simulink model "SimpleTC_SoftwareArch_SoftwareSystem_mapping"  (R2016a)
settings: Solver=FixedStepAuto  StartTime=0.0  StopTime=10.0  RelTol=1e-3
model workspace: external: MAT-File SimpleTC_SoftwareArch_SoftwareSystem_mapping.mat (data not in the file)
libraries: libTLAsserts x6, libAsserts x4
settings Model: Creator=Josef  LastModifiedBy=Josef
settings GRTTargetCC: GeneratePreprocessorConditionals=Use local settings

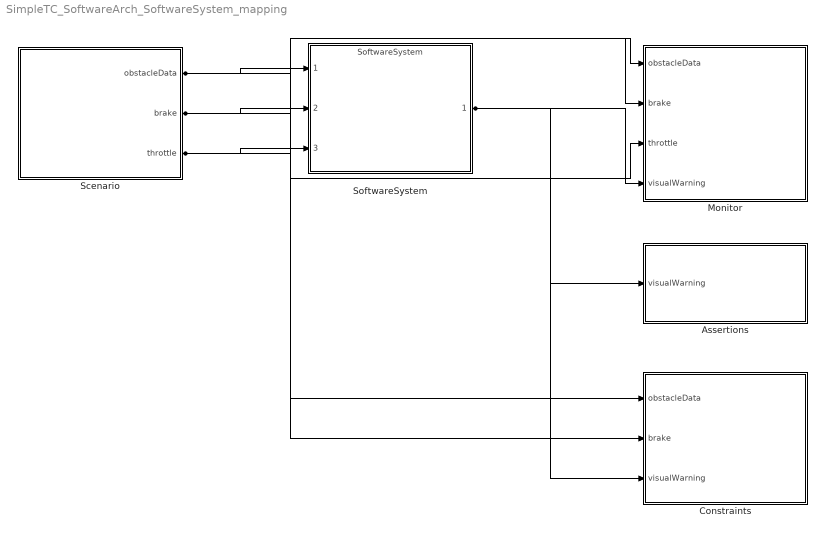
== system SimpleTC_SoftwareArch_SoftwareSystem_mapping ==
  Assertions : Subsystem
  Constraints : Subsystem
  Monitor : Subsystem
  Scenario : Subsystem
  SoftwareSystem : ModelReference  ModelNameDialog=SoftwareSystem  SimulationMode=Normal  ModelReferenceVersion=1.9
  wires:
  Scenario/2(brake) -> SoftwareSystem/2, Monitor/2(brake), Constraints/2(brake)
  Scenario/3(throttle) -> SoftwareSystem/3, Monitor/3(throttle)
  Scenario/1(obstacleData) -> SoftwareSystem/1, Monitor/1(obstacleData), Constraints/1(obstacleData)
  SoftwareSystem/1 -> Monitor/4(visualWarning), Assertions/1(visualWarning), Constraints/3(visualWarning)

== system SimpleTC_SoftwareArch_SoftwareSystem_mapping/Assertions ==
  visualWarning : Inport
  assert_1 : Subsystem
  simout_1 : ToFile  Filename=assert_1.mat  MatrixName=assert_1  SaveFormat=Timeseries
  wires:
  visualWarning/1 -> assert_1/1(visualWarning)
  assert_1/1(assert_1_FAILED) -> simout_1/1

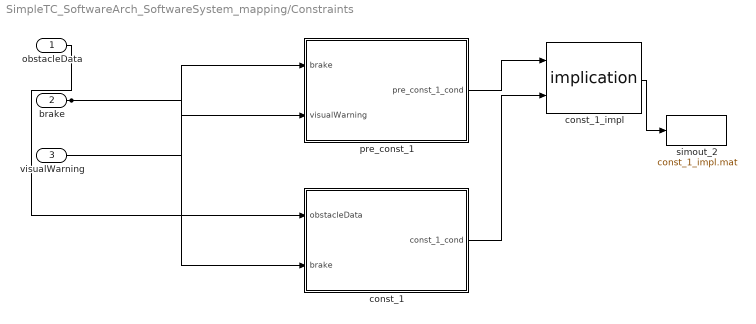
== system SimpleTC_SoftwareArch_SoftwareSystem_mapping/Constraints ==
  obstacleData : Inport
  brake : Inport  Port=2
  visualWarning : Inport  Port=3
  const_1 : Subsystem
  const_1_impl : libAsserts/implication
  pre_const_1 : Subsystem
  simout_2 : ToFile  Filename=const_1_impl.mat  MatrixName=const_1_impl  SaveFormat=Timeseries
  wires:
  brake/1 -> pre_const_1/1(brake), const_1/2(brake)
  visualWarning/1 -> pre_const_1/2(visualWarning)
  obstacleData/1 -> const_1/1(obstacleData)
  pre_const_1/1(pre_const_1_cond) -> const_1_impl/1
  const_1/1(const_1_cond) -> const_1_impl/2
  const_1_impl/1 -> simout_2/1

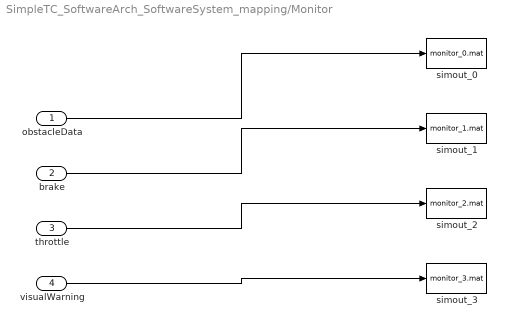
== system SimpleTC_SoftwareArch_SoftwareSystem_mapping/Monitor ==
  obstacleData : Inport
  brake : Inport  Port=2
  throttle : Inport  Port=3
  visualWarning : Inport  Port=4
  simout_0 : ToFile  Filename=monitor_0.mat  MatrixName=obstacleData  SaveFormat=Timeseries
  simout_1 : ToFile  Filename=monitor_1.mat  MatrixName=brake  SaveFormat=Timeseries
  simout_2 : ToFile  Filename=monitor_2.mat  MatrixName=throttle  SaveFormat=Timeseries
  simout_3 : ToFile  Filename=monitor_3.mat  MatrixName=visualWarning  SaveFormat=Timeseries
  wires:
  obstacleData/1 -> simout_0/1
  brake/1 -> simout_1/1
  throttle/1 -> simout_2/1
  visualWarning/1 -> simout_3/1

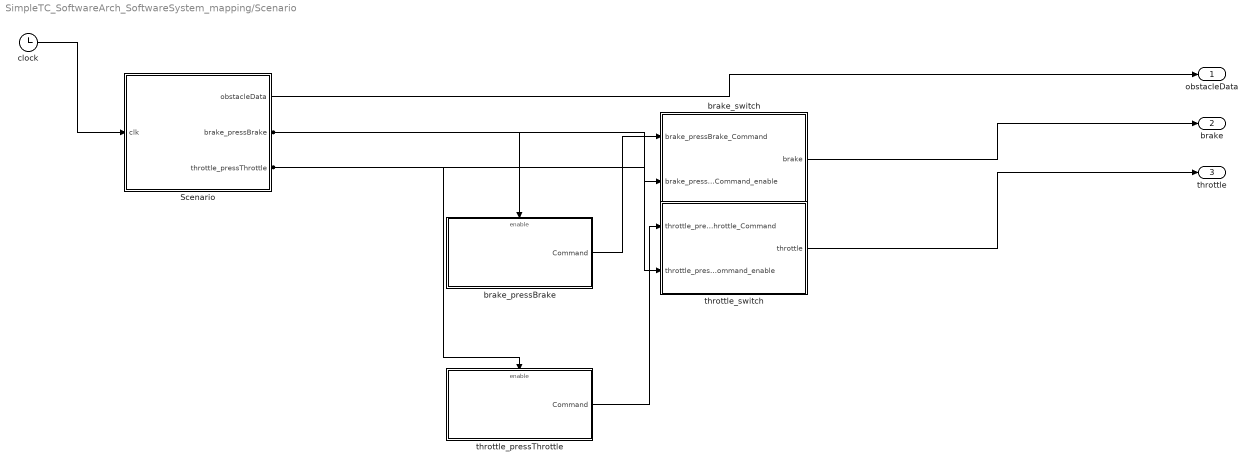
== system SimpleTC_SoftwareArch_SoftwareSystem_mapping/Scenario ==
  Scenario : Stateflow chart  TreatAsAtomicUnit=on
  brake_pressBrake : Subsystem
  brake_switch : Subsystem
  clock : Clock
  throttle_pressThrottle : Subsystem
  throttle_switch : Subsystem
  obstacleData : Outport
  brake : Outport  Port=2
  throttle : Outport  Port=3
  wires:
  brake_switch/1(brake) -> brake/1
  throttle_switch/1(throttle) -> throttle/1
  brake_pressBrake/1(Command) -> brake_switch/1(brake_pressBrake_Command)
  Scenario/2(brake_pressBrake) -> brake_switch/2(brake_pressBrake_Command_enable), brake_pressBrake/Enable
  throttle_pressThrottle/1(Command) -> throttle_switch/1(throttle_pressThrottle_Command)
  Scenario/3(throttle_pressThrottle) -> throttle_switch/2(throttle_pressThrottle_Command_enable), throttle_pressThrottle/Enable
  Scenario/1(obstacleData) -> obstacleData/1
  clock/1 -> Scenario/1(clk)

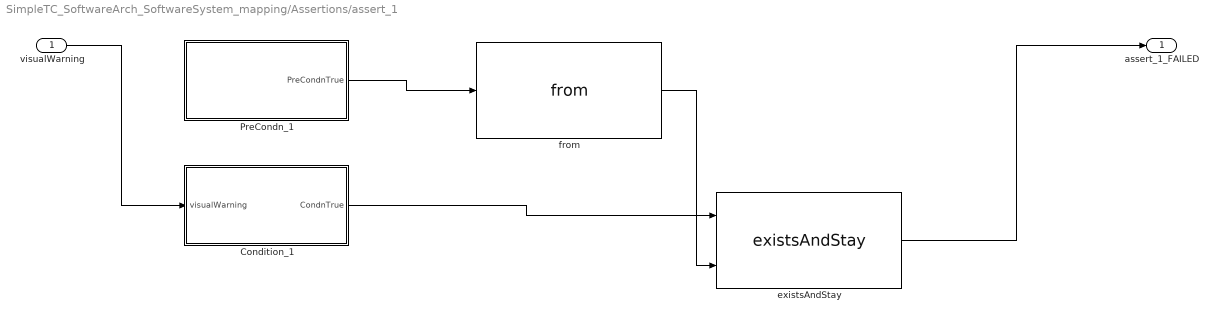
== system SimpleTC_SoftwareArch_SoftwareSystem_mapping/Assertions/assert_1 ==
  visualWarning : Inport
  Condition_1 : Subsystem
  PreCondn_1 : Subsystem
  existsAndStay : libTLAsserts/existsAndStay
  from : libTLAsserts/from
  assert_1_FAILED : Outport
  wires:
  visualWarning/1 -> Condition_1/1(visualWarning)
  PreCondn_1/1(PreCondnTrue) -> from/1
  Condition_1/1(CondnTrue) -> existsAndStay/1
  from/1 -> existsAndStay/2
  existsAndStay/1 -> assert_1_FAILED/1

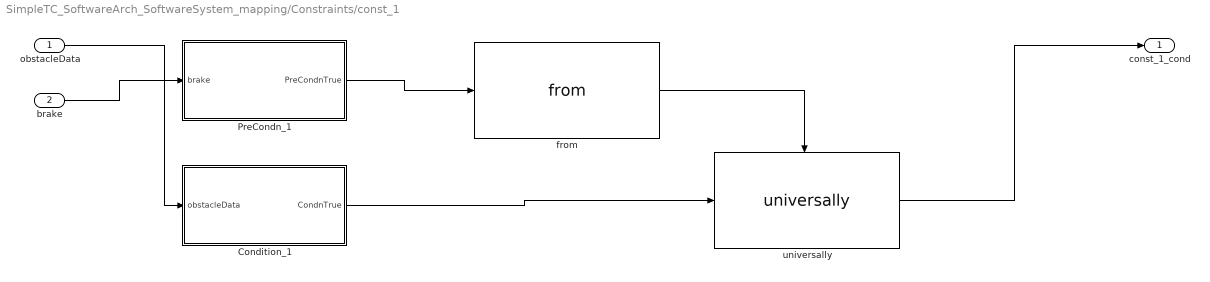
== system SimpleTC_SoftwareArch_SoftwareSystem_mapping/Constraints/const_1 ==
  obstacleData : Inport
  brake : Inport  Port=2
  Condition_1 : Subsystem
  PreCondn_1 : Subsystem
  from : libTLAsserts/from
  universally : libTLAsserts/universally
  const_1_cond : Outport
  wires:
  brake/1 -> PreCondn_1/1(brake)
  obstacleData/1 -> Condition_1/1(obstacleData)
  PreCondn_1/1(PreCondnTrue) -> from/1
  Condition_1/1(CondnTrue) -> universally/1
  from/1 -> universally/Enable
  universally/1 -> const_1_cond/1

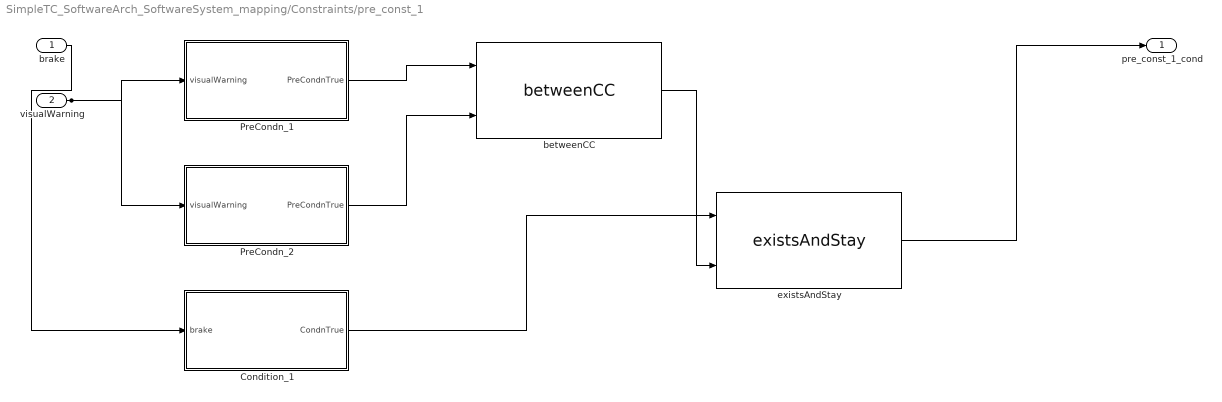
== system SimpleTC_SoftwareArch_SoftwareSystem_mapping/Constraints/pre_const_1 ==
  brake : Inport
  visualWarning : Inport  Port=2
  Condition_1 : Subsystem
  PreCondn_1 : Subsystem
  PreCondn_2 : Subsystem
  betweenCC : libTLAsserts/betweenCC
  existsAndStay : libTLAsserts/existsAndStay
  pre_const_1_cond : Outport
  wires:
  visualWarning/1 -> PreCondn_1/1(visualWarning), PreCondn_2/1(visualWarning)
  brake/1 -> Condition_1/1(brake)
  PreCondn_1/1(PreCondnTrue) -> betweenCC/1
  PreCondn_2/1(PreCondnTrue) -> betweenCC/2
  Condition_1/1(CondnTrue) -> existsAndStay/1
  betweenCC/1 -> existsAndStay/2
  existsAndStay/1 -> pre_const_1_cond/1

== system SimpleTC_SoftwareArch_SoftwareSystem_mapping/Scenario/brake_pressBrake ==
  Enable : EnablePort
  PedalPressed : Constant
  Command : Outport  OutputWhenDisabled=reset  InitialOutput=0
  wires:
  PedalPressed/1 -> Command/1

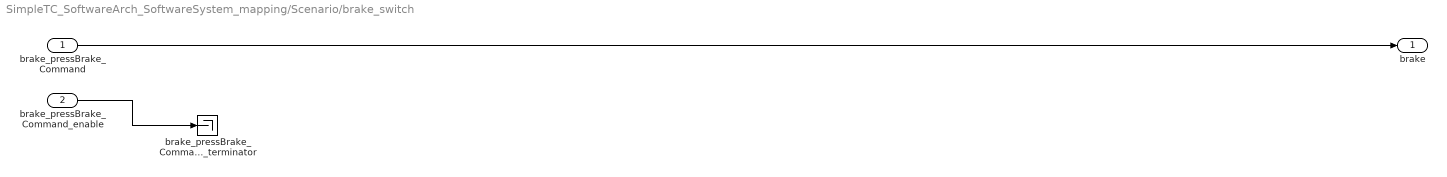
== system SimpleTC_SoftwareArch_SoftwareSystem_mapping/Scenario/brake_switch ==
  brake_pressBrake_Command : Inport
  brake_pressBrake_Command_enable : Inport  Port=2
  brake_pressBrake_Command_terminator : Terminator
  brake : Outport
  wires:
  brake_pressBrake_Command_enable/1 -> brake_pressBrake_Command_terminator/1
  brake_pressBrake_Command/1 -> brake/1

== system SimpleTC_SoftwareArch_SoftwareSystem_mapping/Scenario/throttle_pressThrottle ==
  Enable : EnablePort
  PedalPressed : Constant
  Command : Outport  OutputWhenDisabled=reset  InitialOutput=0
  wires:
  PedalPressed/1 -> Command/1

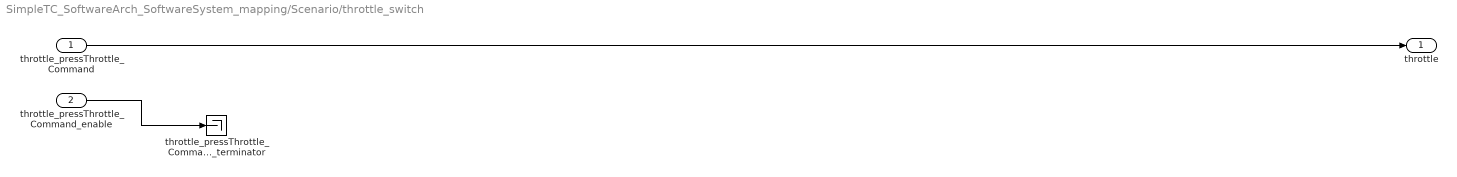
== system SimpleTC_SoftwareArch_SoftwareSystem_mapping/Scenario/throttle_switch ==
  throttle_pressThrottle_Command : Inport
  throttle_pressThrottle_Command_enable : Inport  Port=2
  throttle_pressThrottle_Command_terminator : Terminator
  throttle : Outport
  wires:
  throttle_pressThrottle_Command_enable/1 -> throttle_pressThrottle_Command_terminator/1
  throttle_pressThrottle_Command/1 -> throttle/1

== system SimpleTC_SoftwareArch_SoftwareSystem_mapping/Assertions/assert_1/Condition_1 ==
  visualWarning : Inport
  EqualsExpression_2.0_1.0 : RelationalOperator  Operator===  OutDataTypeStr=boolean
  StringLiteral_1.0_1.0 : Constant
  CondnTrue : Outport
  wires:
  visualWarning/1 -> EqualsExpression_2.0_1.0/1
  StringLiteral_1.0_1.0/1 -> EqualsExpression_2.0_1.0/2
  EqualsExpression_2.0_1.0/1 -> CondnTrue/1

== system SimpleTC_SoftwareArch_SoftwareSystem_mapping/Assertions/assert_1/PreCondn_1 ==
  AnnotatedExpression_2.0_1.0 : RelationalOperator  OutDataTypeStr=boolean
  NumberLiteral_1.0_1.0 : Constant  Value=5
  clock : Clock
  PreCondnTrue : Outport
  wires:
  clock/1 -> AnnotatedExpression_2.0_1.0/1
  NumberLiteral_1.0_1.0/1 -> AnnotatedExpression_2.0_1.0/2
  AnnotatedExpression_2.0_1.0/1 -> PreCondnTrue/1

== system SimpleTC_SoftwareArch_SoftwareSystem_mapping/Constraints/const_1/Condition_1 ==
  obstacleData : Inport
  GreaterExpression_2.0_1.0 : RelationalOperator  Operator=>  OutDataTypeStr=boolean
  NumberLiteral_1.0_1.0 : Constant  Value=100
  CondnTrue : Outport
  wires:
  obstacleData/1 -> GreaterExpression_2.0_1.0/1
  NumberLiteral_1.0_1.0/1 -> GreaterExpression_2.0_1.0/2
  GreaterExpression_2.0_1.0/1 -> CondnTrue/1

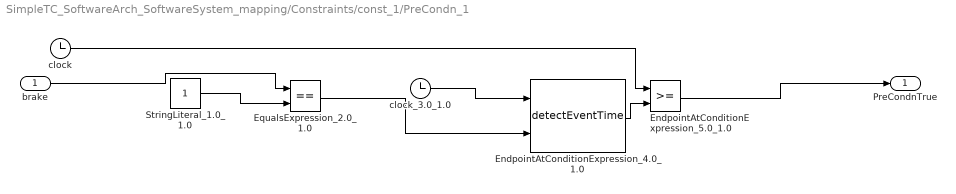
== system SimpleTC_SoftwareArch_SoftwareSystem_mapping/Constraints/const_1/PreCondn_1 ==
  brake : Inport
  EndpointAtConditionExpression_4.0_1.0 : libAsserts/detectEventTime
  EndpointAtConditionExpression_5.0_1.0 : RelationalOperator  OutDataTypeStr=boolean
  EqualsExpression_2.0_1.0 : RelationalOperator  Operator===  OutDataTypeStr=boolean
  StringLiteral_1.0_1.0 : Constant
  clock : Clock
  clock_3.0_1.0 : Clock
  PreCondnTrue : Outport
  wires:
  brake/1 -> EqualsExpression_2.0_1.0/1
  StringLiteral_1.0_1.0/1 -> EqualsExpression_2.0_1.0/2
  clock_3.0_1.0/1 -> EndpointAtConditionExpression_4.0_1.0/1
  EqualsExpression_2.0_1.0/1 -> EndpointAtConditionExpression_4.0_1.0/2
  clock/1 -> EndpointAtConditionExpression_5.0_1.0/1
  EndpointAtConditionExpression_4.0_1.0/1 -> EndpointAtConditionExpression_5.0_1.0/2
  EndpointAtConditionExpression_5.0_1.0/1 -> PreCondnTrue/1

== system SimpleTC_SoftwareArch_SoftwareSystem_mapping/Constraints/pre_const_1/Condition_1 ==
  brake : Inport
  EqualsExpression_2.0_1.0 : RelationalOperator  Operator===  OutDataTypeStr=boolean
  StringLiteral_1.0_1.0 : Constant
  CondnTrue : Outport
  wires:
  brake/1 -> EqualsExpression_2.0_1.0/1
  StringLiteral_1.0_1.0/1 -> EqualsExpression_2.0_1.0/2
  EqualsExpression_2.0_1.0/1 -> CondnTrue/1

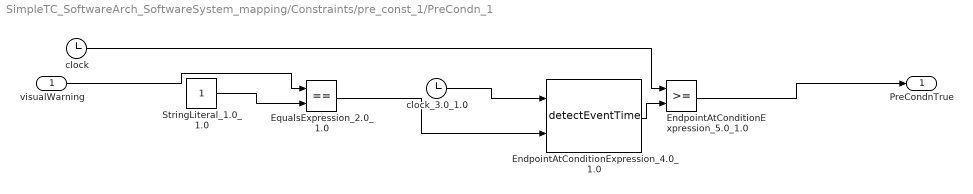
== system SimpleTC_SoftwareArch_SoftwareSystem_mapping/Constraints/pre_const_1/PreCondn_1 ==
  visualWarning : Inport
  EndpointAtConditionExpression_4.0_1.0 : libAsserts/detectEventTime
  EndpointAtConditionExpression_5.0_1.0 : RelationalOperator  OutDataTypeStr=boolean
  EqualsExpression_2.0_1.0 : RelationalOperator  Operator===  OutDataTypeStr=boolean
  StringLiteral_1.0_1.0 : Constant
  clock : Clock
  clock_3.0_1.0 : Clock
  PreCondnTrue : Outport
  wires:
  visualWarning/1 -> EqualsExpression_2.0_1.0/1
  StringLiteral_1.0_1.0/1 -> EqualsExpression_2.0_1.0/2
  clock_3.0_1.0/1 -> EndpointAtConditionExpression_4.0_1.0/1
  EqualsExpression_2.0_1.0/1 -> EndpointAtConditionExpression_4.0_1.0/2
  clock/1 -> EndpointAtConditionExpression_5.0_1.0/1
  EndpointAtConditionExpression_4.0_1.0/1 -> EndpointAtConditionExpression_5.0_1.0/2
  EndpointAtConditionExpression_5.0_1.0/1 -> PreCondnTrue/1

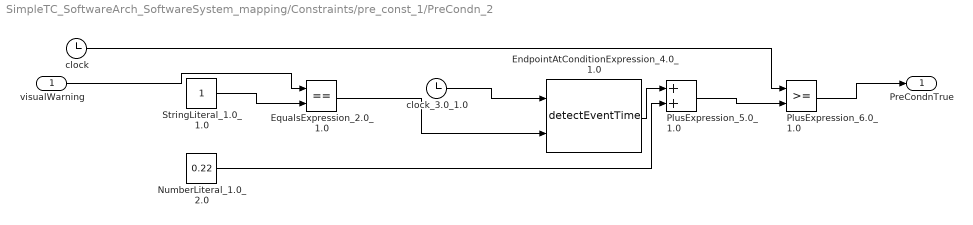
== system SimpleTC_SoftwareArch_SoftwareSystem_mapping/Constraints/pre_const_1/PreCondn_2 ==
  visualWarning : Inport
  EndpointAtConditionExpression_4.0_1.0 : libAsserts/detectEventTime
  EqualsExpression_2.0_1.0 : RelationalOperator  Operator===  OutDataTypeStr=boolean
  NumberLiteral_1.0_2.0 : Constant  Value=0.22
  PlusExpression_5.0_1.0 : Sum
  PlusExpression_6.0_1.0 : RelationalOperator  OutDataTypeStr=boolean
  StringLiteral_1.0_1.0 : Constant
  clock : Clock
  clock_3.0_1.0 : Clock
  PreCondnTrue : Outport
  wires:
  visualWarning/1 -> EqualsExpression_2.0_1.0/1
  StringLiteral_1.0_1.0/1 -> EqualsExpression_2.0_1.0/2
  clock_3.0_1.0/1 -> EndpointAtConditionExpression_4.0_1.0/1
  EqualsExpression_2.0_1.0/1 -> EndpointAtConditionExpression_4.0_1.0/2
  EndpointAtConditionExpression_4.0_1.0/1 -> PlusExpression_5.0_1.0/1
  NumberLiteral_1.0_2.0/1 -> PlusExpression_5.0_1.0/2
  clock/1 -> PlusExpression_6.0_1.0/1
  PlusExpression_5.0_1.0/1 -> PlusExpression_6.0_1.0/2
  PlusExpression_6.0_1.0/1 -> PreCondnTrue/1

== stateflow chart SimpleTC_SoftwareArch_SoftwareSystem_mapping/Scenario/Scenario ==
  state Act_Subject [parallel]
    settings: executionOrder=1
    state Act_Subject_Step1
      entry: brake_pressBrake = 0;
      entry: throttle_pressThrottle = 1;
    (default) -> Act_Subject_Step1
  state Act_Obstacle [parallel]
    settings: executionOrder=2
    state Act_Obstacle_Step1
      entry: obstacleData = 50;
    state Act_Obstacle_Step2
      entry: obstacleData = obstacleData - 10;
      entry: Act_Obstacle_Step2_stpClk = clk;
    state Act_Obstacle_Step3
    (default) -> Act_Obstacle_Step1
    Act_Obstacle_Step1 -> Act_Obstacle_Step2 : [clk > 5]
    Act_Obstacle_Step2 -> Act_Obstacle_Step3 : [clk - Act_Obstacle_Step2_stpClk > 1]
    Act_Obstacle_Step3 -> Act_Obstacle_Step2
  data: clk input; obstacleData output; brake_pressBrake output; throttle_pressThrottle output; Act_Obstacle_Step2_stpClk local
